simulink model "blockdemo"  (Simulink 6.3)
settings: Solver=ode45  StartTime=0.0  StopTime=79  RelTol=1e-3
InitFcn:
  | %% DSPBuilder Start
  | alt_dspbuilder_update_model(bdroot)
  | %% DSPBuilder End
libraries: allblocks_alteradspbuilder2 x6
settings Model: Creator=cpurcell  LastModifiedBy=delphick
settings DebuggingCC: MultiTaskDSMMsg=error

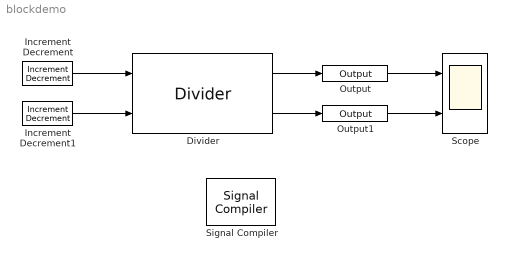
== system blockdemo ==
  Divider : allblocks_alteradspbuilder2/Divider  BusType=Signed Fractional  bwl=8  bwr=2  pipeline=1  use_ena=off  use_aclr=off
  Increment Decrement : allblocks_alteradspbuilder2/Increment Decrement  BusType=Signed Fractional  bwl=8  bwr=2  SpecifyClock=off  clr_value=0  direction=Increment  phase_selection=1  use_ena=off  use_sclr=off
  Increment Decrement1 : allblocks_alteradspbuilder2/Increment Decrement  BusType=Signed Fractional  bwl=8  bwr=2  SpecifyClock=off  clr_value=20  direction=Decrement  phase_selection=1  use_ena=off  use_sclr=off
  Output : allblocks_alteradspbuilder2/Output  iofile=C:\workspace_clean\Documentation\DesignExamples\Tutorials\UnitBlocks\Arithmetic\Divider\tb_blockdemo\blockdemo_Output.capture  BusType=Inferred  bwl=10  bwr=0  PORTTYPE=Output
  Output1 : allblocks_alteradspbuilder2/Output  iofile=C:\workspace_clean\Documentation\DesignExamples\Tutorials\UnitBlocks\Arithmetic\Divider\tb_blockdemo\blockdemo_Output1.capture  BusType=Inferred  bwl=8  bwr=2  PORTTYPE=Output
  Scope : Scope  NumInputPorts=2
      settings: TimeRange=80  YMin=-1~-0.5  YMax=41~10.5
  Signal Compiler : allblocks_alteradspbuilder2/Signal Compiler  DeviceFamily=Stratix IV  DeviceName=AUTO  EnableSignalTap=off  SignalTapDepth=128  UseBoardBlock=off  StpUseDefaultClock=on  StpClock=clock
  wires:
  Increment Decrement/1 -> Divider/1
  Increment Decrement1/1 -> Divider/2
  Divider/1 -> Output/1
  Divider/2 -> Output1/1
  Output/1 -> Scope/1
  Output1/1 -> Scope/2
